simulink model "VBattery_harness"  (Simulink 7.7)
settings: Solver=FixedStepDiscrete  StartTime=0.0  StopTime=100.0  FixedStep=.1  RelTol=1e-3
PostLoadFcn:
  | load Vbattery.mat
InitFcn:
  | if signalbuilder('VBattery_harness/Signal_Builder','activegroup') == 1
  |   CD_VBATTERY_FUNCTION.DataType = 'uint8';
  |   CD_VBATTERY_FUNCTION.Value = 255;
  |   CD_ALTERNATOR_FUNCTION.DataType = 'uint8';
  |   CD_ALTERNATOR_FUNCTION.Value = 255;
  | elseif signalbuilder('VBattery_harness/Signal_Builder','activegroup') == 2
  |   CD_ALTERNATOR_FUNCTION.DataType = 'uint8';
  |   CD_ALTERNATOR_FUNCTION.Value = 255;
  |   CD_VBATTERY_FUNCTION.DataType = 'uint8';
  |   CD_VBATTERY_FUNCTION.Value = 0;
  | else
  |   CD_VBATTERY_FUNCTION.DataType = 'uint8';
  |   CD_VBATTERY_FUNCTION.Value = 0;
  |   CD_ALTERNATOR_FUNCTION.DataType = 'uint8';
  |   CD_ALTERNATOR_FUNCTION.Value = 0;
  | end
undefined symbols (not defined in the file): CD_PRECISION_REF_NOMINAL_VALUE, CD_VBATTERY_FILTER_DISPLAY_GAIN, CD_VBATTERY_FILTER_GAIN, CD_VBATTERY_GAIN, sigbuilder_block, srate100
settings Model: Creator=smindema  LastModifiedBy=aliebel  RecordCoverage=on  CovMetricSettings=dcw  CovCumulativeReport=on
settings DataIOCC: SaveFormat=Structure
settings OptimizationCC: InlineParams=on  InitFltsAndDblsToZero=on  EfficientFloat2IntCast=on  OptimizeModelRefInitCode=on
settings DebuggingCC: SaveWithParameterizedLinksMsg=none  SignalResolutionControl=TryResolveAllWithWarning  MultiTaskDSMMsg=warning  MultiTaskCondExecSysMsg=none  StrictBusMsg=Warning
settings HardwareCC: ProdBitPerInt=16  ProdBitPerPointer=16  ProdIntDivRoundTo=Floor  ProdEndianess=BigEndian  ProdWordSize=16  ProdHWDeviceType=Motorola HC12  TargetHWDeviceType=32-bit Generic  ProdEqTarget=off
settings RTWCC: SystemTargetFile=ert.tlc  GenCodeOnly=on  TemplateMakefile=ert_default_tmf  Description=Real-Time Workshop Embedded Coder (no auto configuration)  ProcessScript=ert_make_rtw_hook  IncludeERTFirstTime=on
settings CodeAppCC: IgnoreCustomStorageClasses=off
settings ERTTargetCC: TargetFcnLib=ansi_tfl_tmw.mat  FunctionExecutionProfile=off  MultiwordLength=2048  GenerateSampleERTMain=on  IncludeMdlTerminateFcn=off  SupportNonFinite=off  SupportComplex=off  PurelyIntegerCode=on  InlinedParameterPlacement=NonHierarchical  ERTCustomFileTemplate=example_file_process.tlc  ConvertIfToSwitch=off

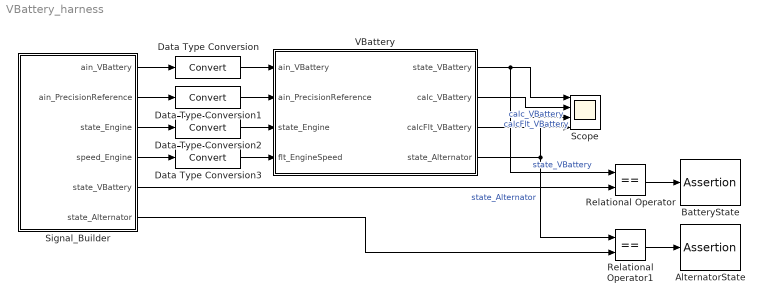
== system VBattery_harness ==
  AlternatorState : Assertion  Enabled=off
  BatteryState : Assertion  Enabled=off
  Data Type Conversion{,1..3} (4 alike) : DataTypeConversion
  Relational Operator : RelationalOperator  Operator===  OutDataTypeStr=boolean
  Relational Operator1 : RelationalOperator  Operator===  OutDataTypeStr=boolean
  Scope : Scope  NumInputPorts=4
      settings: TimeRange=100  YMin=8~14.5~14.5~8  YMax=11~21~21~10  MaxDataPoints=100000
  Signal_Builder : Subsystem  Tag=STV Subsys  LoadFcn=sigbuilder_block('load');  StartFcn=sigbuilder_block('start');  StopFcn=sigbuilder_block('stop');  ClipboardFcn=sigbuilder_block('clipboard');  mask(Sigbuilder block){}
      mask help: Sigbuilder GUI
      mask init:
      | if ~strcmp(get_param(bdroot(gcbh),'SimulationStatus'),'stopped') tuvar = sigbuilder_block('maskInit'); end
      settings: CopyFcn=sigbuilder_block('copy');  DeleteFcn=sigbuilder_block('delete');  ModelCloseFcn=sigbuilder_block('modelClose');  PreSaveFcn=sigbuilder_block('preSave');  NameChangeFcn=sigbuilder_block('namechange');  OpenFcn=sigbuilder_block('open',[50.25 223.5 1137 507 ]);  CloseFcn=sigbuilder_block('close');
      mask Display: plot(0,0,100,100,[10,10,40,40,10],[80,20,20,80,80],[40,10],[50,50], [40,27,10],[65,72,56],[40,25,25,10],[28,28,43,43]);
  VBattery : Subsystem  TreatAsAtomicUnit=on  SystemSampleTime=srate100  RTWFileName=mod_Inputs
      settings: RTWSystemCode=Function  RTWFcnNameOpts=Use subsystem name  RTWFileNameOpts=User specified
  wires:
  Signal_Builder/1(ain_VBattery) -> Data Type Conversion/1
  Data Type Conversion/1 -> VBattery/1(ain_VBattery)
  Data Type Conversion1/1 -> VBattery/2(ain_PrecisionReference)
  VBattery/1(state_VBattery) -> Scope/1, Relational Operator/1  "state_VBattery"
  VBattery/2(calc_VBattery) -> Scope/2  "calc_VBattery"
  VBattery/3(calcFlt_VBattery) -> Scope/3  "calcFlt_VBattery"
  Data Type Conversion2/1 -> VBattery/3(state_Engine)
  Signal_Builder/5(state_VBattery) -> Relational Operator/2
  Relational Operator/1 -> BatteryState/1
  Signal_Builder/4(speed_Engine) -> Data Type Conversion3/1
  Data Type Conversion3/1 -> VBattery/4(flt_EngineSpeed)
  Relational Operator1/1 -> AlternatorState/1
  VBattery/4(state_Alternator) -> Relational Operator1/1, Scope/4  "state_Alternator"
  Signal_Builder/6(state_Alternator) -> Relational Operator1/2
  Signal_Builder/2(ain_PrecisionReference) -> Data Type Conversion1/1
  Signal_Builder/3(state_Engine) -> Data Type Conversion2/1

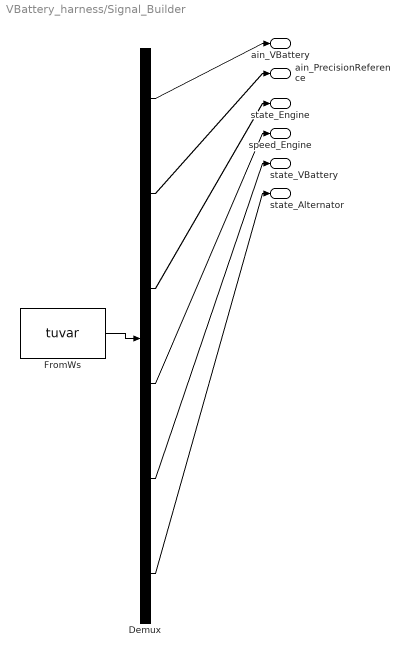
== system VBattery_harness/Signal_Builder ==
  Demux : Demux  Tag=STV Demux  Outputs=6
  FromWs : FromWorkspace  Tag=STV FromWs  VariableName=tuvar  SampleTime=0  SigBuilderData=DataTag0  VnvData=DataTag1
      SigBuilderData=|
      | common.afterFinalStr = 'Extrapolate'
      | common.sampleTime = 0
      | dataSet(1).timeRange = [0 100]
      | dataSet(1).name = 'T1-NONFUNC'
      | dataSet(2).timeRange = [0 100]
      | dataSet(2).name = 'T2-ALT NONFUNC'
      | dataSet(3).timeRange = [0 100]
      | dataSet(3).name = 'ALT_LOW'
      | dataSet(4).timeRange = [0 100]
      | dataSet(4).name = 'OORL'
      | dataSet(5).timeRange = [0 100]
      | dataSet(5).name = 'LOW'
      | dataSet(6).timeRange = [0 100]
      | dataSet(6).name = 'HIGH'
      | dataSet(7).timeRange = [0 100]
      | dataSet(7).name = 'NORMAL'
      | dataSet(8).timeRange = [0 100]
      | dataSet(8).name = 'HIGH2'
      | dataSet(9).timeRange = [0 100]
      | dataSet(9).name = 'HIGH3'
      | dataSet(10).timeRange = [0 100]
      | dataSet(10).name = 'ALT_HIGH'
      | sbobj.Groups(1).Name = 'T1-NONFUNC'
      | sbobj.Groups(1).Signals(1).Name = 'ain_VBattery'
      | sbobj.Groups(1).Signals(1).XData = [0 10 10 10.3 10.3 10.9 10.9 21.9 21.9 22.2 22.2 29.9 29.9 30.2 30.2 30.5 30.5 31.1 31.1 31.5 31.5 38.2 38.2 38.5 38.5 44 44 45.6 45.6 45.7 45.7 48 48 48.3 48.3 53.5 53.5 53.7 53.7 60 60 66.4 66.4 69.9 69.9 79.8 79.8 89.9 89.9 100]
      | sbobj.Groups(1).Signals(1).YData = [500 500 298 298 500 500 298 298 500 500 298 298 226 226 500 500 226 226 300 300 226 226 390 332 226 226 500 500 226 226 500 500 300 300 500 500 300 300 500 500 296 296 502 502 224 224 298 298 500 500]
      | sbobj.Groups(1).Signals(2).Name = 'ain_PrecisionReference'
      | sbobj.Groups(1).Signals(2).XData = [0 100]
      | sbobj.Groups(1).Signals(2).YData = [509 509]
      | sbobj.Groups(1).Signals(3).Name = 'state_Engine'
      | sbobj.Groups(1).Signals(3).XData = [0 50 50 100]
      | sbobj.Groups(1).Signals(3).YData = [1 1 2 2]
      | sbobj.Groups(1).Signals(4).Name = 'speed_Engine'
      | sbobj.Groups(1).Signals(4).XData = [0 8.6 8.6 53.2 53.2 65.2 65.2 100]
      | sbobj.Groups(1).Signals(4).YData = [0 0 1500 1500 0 0 1500 1500]
      | sbobj.Groups(1).Signals(5).Name = 'state_VBattery'
      | sbobj.Groups(1).Signals(5).XData = [0 100]
      | sbobj.Groups(1).Signals(5).YData = [8 8]
      | sbobj.Groups(1).Signals(6).Name = 'state_Alternator'
      | sbobj.Groups(1).Signals(6).XData = [0 100]
      | sbobj.Groups(1).Signals(6).YData = [8 8]
      | sbobj.Groups(2).Name = 'T2-ALT NONFUNC'
      | sbobj.Groups(2).Signals(1).Name = 'ain_VBattery'
      | sbobj.Groups(2).Signals(1).XData = [0 10 10 10.3 10.3 10.9 10.9 21.9 21.9 22.2 22.2 29.9 29.9 30.2 30.2 30.5 30.5 31.1 31.1 31.5 31.5 38.2 38.2 38.5 38.5 45.9 47.4 47.4 53.5 53.5 53.7 53.7 60 60 66.4 66.4 69.9 69.9 79.8 79.8 89.9 89.9 100]
      | sbobj.Groups(2).Signals(1).YData = [500 500 298 298 500 500 298 298 500 500 298 298 226 226 500 500 226 226 300 300 226 226 390 332 300 300 300 630 630 300 300 595 595 296 296 502 502 224 224 298 298 500 500]
      | sbobj.Groups(2).Signals(2).Name = 'ain_PrecisionReference'
      | sbobj.Groups(2).Signals(2).XData = [0 100]
      | sbobj.Groups(2).Signals(2).YData = [509 509]
      | sbobj.Groups(2).Signals(3).Name = 'state_Engine'
      | sbobj.Groups(2).Signals(3).XData = [0 50 50 100]
      | sbobj.Groups(2).Signals(3).YData = [1 1 2 2]
      | sbobj.Groups(2).Signals(4).Name = 'speed_Engine'
      | sbobj.Groups(2).Signals(4).XData = [0 8.6 8.6 34.8 35.2 53.2 53.2 65.2 65.2 100]
      | sbobj.Groups(2).Signals(4).YData = [0 0 1500 1500 1500 1500 0 0 1500 1500]
      | sbobj.Groups(2).Signals(5).Name = 'state_VBattery'
      | sbobj.Groups(2).Signals(5).XData = [0 12.4 12.4 32.2 32.2 38.9 38.9 48 48 48.9 48.9 55.6 60.6 60.6 61.9 61.9 71.7 71.7 100]
      | sbobj.Groups(2).Signals(5).YData = [8 8 9 9 14 14 9 9 8 8 10 10 10 8 8 9 9 14 14]
      | sbobj.Groups(2).Signals(6).Name = 'state_Alternator'
      | sbobj.Groups(2).Signals(6).XData = [0 100]
      | sbobj.Groups(2).Signals(6).YData = [8 8]
      | sbobj.Groups(3).Name = 'ALT_LOW'
      | sbobj.Groups(3).Signals(1).Name = 'ain_VBattery'
      | sbobj.Groups(3).Signals(1).XData = [0 10 10 10.3 10.3 10.9 10.9 21.9 21.9 22.2 22.2 29.9 29.9 30.2 30.2 30.5 30.5 31.1 31.1 31.5 31.5 38.2 38.2 38.5 38.5 42.4 42.4 53.1 53.1 53.5 53.5 53.7 53.7 60 60 66.4 66.4 69.9 69.9 79.8 79.8 89.9 89.9 100]
      | sbobj.Groups(3).Signals(1).YData = [500 500 298 298 500 500 298 298 500 500 298 298 226 226 500 500 226 226 300 300 226 226 390 332 226 226 360 360 500 500 300 300 500 500 296 296 502 502 224 224 298 298 500 500]
      | sbobj.Groups(3).Signals(2).Name = 'ain_PrecisionReference'
      | sbobj.Groups(3).Signals(2).XData = [0 100]
      | sbobj.Groups(3).Signals(2).YData = [509 509]
      | sbobj.Groups(3).Signals(3).Name = 'state_Engine'
      | sbobj.Groups(3).Signals(3).XData = [0 50 50 70 70 100]
      | sbobj.Groups(3).Signals(3).YData = [1 1 2 2 3 3]
      | sbobj.Groups(3).Signals(4).Name = 'speed_Engine'
      | sbobj.Groups(3).Signals(4).XData = [0 8.6 8.6 22.7 22.7 26.6 26.6 42 42 47.3 47.3 53.2 53.2 69 69 100]
      | sbobj.Groups(3).Signals(4).YData = [0 0 1500 1500 20 20 1500 1500 0 0 1500 1500 0 0 1500 1500]
      | sbobj.Groups(3).Signals(5).Name = 'state_VBattery'
      | sbobj.Groups(3).Signals(5).XData = [0 12.4 23.3 23.3 32.2 32.2 43.2 43.2 45.7 45.7 61.6 61.6 70.7 70.7 71.7 71.7 81 81 100]
      | sbobj.Groups(3).Signals(5).YData = [8 8 8 9 9 14 14 9 9 8 8 9 9 8 8 14 14 8 8]
      | sbobj.Groups(3).Signals(6).Name = 'state_Alternator'
      | sbobj.Groups(3).Signals(6).XData = [0 11.7 11.7 23.3 23.3 47.8 47.8 53.7 53.7 70.7 70.7 71.7 71.7 81 81 91.1 91.1 100]
      | sbobj.Groups(3).Signals(6).YData = [8 8 9 9 8 8 9 9 8 8 9 9 8 8 9 9 8 8]
      | sbobj.Groups(4).Name = 'OORL'
      | sbobj.Groups(4).Signals(1).Name = 'ain_VBattery'
      | sbobj.Groups(4).Signals(1).XData = [0 29.9 29.9 30.6 30.6 40 40 48.3 48.3 52.2 52.2 78 78 87 87 94 94 94.7 94.7 100]
      | sbobj.Groups(4).Signals(1).YData = [500 500 0 0 500 500 4 4 495 495 34 34 500 500 38 38 500 500 38 38]
      | sbobj.Groups(4).Signals(2).Name = 'ain_PrecisionReference'
      | sbobj.Groups(4).Signals(2).XData = [0 100]
      | sbobj.Groups(4).Signals(2).YData = [509 509]
      | sbobj.Groups(4).Signals(3).Name = 'state_Engine'
      | sbobj.Groups(4).Signals(3).XData = [0 37.6 37.6 67.6 67.6 100]
      | sbobj.Groups(4).Signals(3).YData = [1 1 2 2 1 1]
      | sbobj.Groups(4).Signals(4).Name = 'speed_Engine'
      | sbobj.Groups(4).Signals(4).XData = [0 100]
      | sbobj.Groups(4).Signals(4).YData = [0 0]
      | sbobj.Groups(4).Signals(5).Name = 'state_VBattery'
      | sbobj.Groups(4).Signals(5).XData = [0 41.1 41.1 79.3 79.3 88.2 88.2 100]
      | sbobj.Groups(4).Signals(5).YData = [8 8 22 22 8 8 22 22]
      | sbobj.Groups(4).Signals(6).Name = 'state_Alternator'
      | sbobj.Groups(4).Signals(6).XData = [0 100]
      | sbobj.Groups(4).Signals(6).YData = [8 8]
      | sbobj.Groups(5).Name = 'LOW'
      | sbobj.Groups(5).Signals(1).Name = 'ain_VBattery'
      | sbobj.Groups(5).Signals(1).XData = [0 10 10 10.3 10.3 10.9 10.9 21.9 21.9 22.2 22.2 29.9 29.9 30.2 30.2 30.5 30.5 31.1 31.1 31.5 31.5 38.2 38.2 38.5 38.5 44 44 45.6 45.6 45.7 45.7 48 48 48.3 48.3 53.5 53.5 53.7 53.7 60 60 66.4 66.4 69.9 69.9 79.8 79.8 89.9 89.9 100]
      | sbobj.Groups(5).Signals(1).YData = [500 500 298 298 500 500 298 298 500 500 298 298 226 226 500 500 226 226 300 300 226 226 390 332 226 226 500 500 226 226 500 500 300 300 500 500 300 300 500 500 296 296 502 502 224 224 298 298 500 500]
      | sbobj.Groups(5).Signals(2).Name = 'ain_PrecisionReference'
      | sbobj.Groups(5).Signals(2).XData = [0 100]
      | sbobj.Groups(5).Signals(2).YData = [509 509]
      | sbobj.Groups(5).Signals(3).Name = 'state_Engine'
      | sbobj.Groups(5).Signals(3).XData = [0 50 50 100]
      | sbobj.Groups(5).Signals(3).YData = [1 1 2 2]
      | sbobj.Groups(5).Signals(4).Name = 'speed_Engine'
      | sbobj.Groups(5).Signals(4).XData = [0 91.7 91.7 92 92 100]
      | sbobj.Groups(5).Signals(4).YData = [0 0 1600 1600 0 0]
      | sbobj.Groups(5).Signals(5).Name = 'state_VBattery'
      | sbobj.Groups(5).Signals(5).XData = [0 12.4 12.4 32.2 32.2 44.9 44.9 61.6 61.6 71.7 71.7 83.4 86.3 92.3 92.3 100]
      | sbobj.Groups(5).Signals(5).YData = [8 8 9 9 14 14 8 8 9 9 14 14 14 14 8 8]
      | sbobj.Groups(5).Signals(6).Name = 'state_Alternator'
      | sbobj.Groups(5).Signals(6).XData = [0 100]
      | sbobj.Groups(5).Signals(6).YData = [8 8]
      | sbobj.Groups(6).Name = 'HIGH'
      | sbobj.Groups(6).Signals(1).Name = 'ain_VBattery'
      | sbobj.Groups(6).Signals(1).XData = [0 10 10 10.3 10.3 10.9 10.9 16 16 16.5 16.5 21.9 21.9 22.2 22.2 29.9 29.9 30.2 30.2 30.4 30.4 30.7 30.7 30.9 30.9 38 38 38.1 38.1 44 44 45.6 45.6 45.7 45.7 48 48 48.3 48.3 53.5 53.5 53.7 53.7 60 60 69.9 69.9 79.8 79.8 89.9 89.9 100]
      | sbobj.Groups(6).Signals(1).YData = [500 500 630 630 500 500 570 570 738 738 570 570 500 500 572 572 700 700 500 500 700 700 625 625 700 700 500 500 700 700 500 500 700 700 500 500 620 625 500 500 630 630 500 500 562 562 700 700 556 556 500 500]
      | sbobj.Groups(6).Signals(2).Name = 'ain_PrecisionReference'
      | sbobj.Groups(6).Signals(2).XData = [0 100]
      | sbobj.Groups(6).Signals(2).YData = [509 509]
      | sbobj.Groups(6).Signals(3).Name = 'state_Engine'
      | sbobj.Groups(6).Signals(3).XData = [0 50 50 100]
      | sbobj.Groups(6).Signals(3).YData = [1 1 2 2]
      | sbobj.Groups(6).Signals(4).Name = 'speed_Engine'
      | sbobj.Groups(6).Signals(4).XData = [0 100]
      | sbobj.Groups(6).Signals(4).YData = [0 0]
      | sbobj.Groups(6).Signals(5).Name = 'state_VBattery'
      | sbobj.Groups(6).Signals(5).XData = [0 11.8 11.8 32.3 32.3 44.6 44.6 46.5 46.5 61.4 61.4 71.8 71.8 80.5 80.5 90.9 90.9 100]
      | sbobj.Groups(6).Signals(5).YData = [8 8 10 10 11 11 10 10 8 8 10 10 11 11 10 10 8 8]
      | sbobj.Groups(6).Signals(6).Name = 'state_Alternator'
      | sbobj.Groups(6).Signals(6).XData = [0 100]
      | sbobj.Groups(6).Signals(6).YData = [8 8]
      | sbobj.Groups(7).Name = 'NORMAL'
      | sbobj.Groups(7).Signals(1).Name = 'ain_VBattery'
      | sbobj.Groups(7).Signals(1).XData = [0 100]
      | sbobj.Groups(7).Signals(1).YData = [498 498]
      | sbobj.Groups(7).Signals(2).Name = 'ain_PrecisionReference'
      | sbobj.Groups(7).Signals(2).XData = [0 100]
      | sbobj.Groups(7).Signals(2).YData = [509 509]
      | sbobj.Groups(7).Signals(3).Name = 'state_Engine'
      | sbobj.Groups(7).Signals(3).XData = [0 50 50 100]
      | sbobj.Groups(7).Signals(3).YData = [1 1 2 2]
      | sbobj.Groups(7).Signals(4).Name = 'speed_Engine'
      | sbobj.Groups(7).Signals(4).XData = [0 100]
      | sbobj.Groups(7).Signals(4).YData = [0 0]
      | sbobj.Groups(7).Signals(5).Name = 'state_VBattery'
      | sbobj.Groups(7).Signals(5).XData = [0 100]
      | sbobj.Groups(7).Signals(5).YData = [8 8]
      | sbobj.Groups(7).Signals(6).Name = 'state_Alternator'
      | sbobj.Groups(7).Signals(6).XData = [0 100]
      | sbobj.Groups(7).Signals(6).YData = [8 8]
      | sbobj.Groups(8).Name = 'HIGH2'
      | sbobj.Groups(8).Signals(1).Name = 'ain_VBattery'
      | sbobj.Groups(8).Signals(1).XData = [0 20 20 60 60 100]
      | sbobj.Groups(8).Signals(1).YData = [498 498 610 610 0 0]
      | sbobj.Groups(8).Signals(2).Name = 'ain_PrecisionReference'
      | sbobj.Groups(8).Signals(2).XData = [0 100]
      | sbobj.Groups(8).Signals(2).YData = [509 509]
      | sbobj.Groups(8).Signals(3).Name = 'state_Engine'
      | sbobj.Groups(8).Signals(3).XData = [0 50 50 100]
      | sbobj.Groups(8).Signals(3).YData = [1 1 2 2]
      | sbobj.Groups(8).Signals(4).Name = 'speed_Engine'
      | sbobj.Groups(8).Signals(4).XData = [0 100]
      | sbobj.Groups(8).Signals(4).YData = [0 0]
      | sbobj.Groups(8).Signals(5).Name = 'state_VBattery'
      | sbobj.Groups(8).Signals(5).XData = [0 20.8 20.8 61.3 61.3 100]
      | sbobj.Groups(8).Signals(5).YData = [8 8 10 10 22 22]
      | sbobj.Groups(8).Signals(6).Name = 'state_Alternator'
      | sbobj.Groups(8).Signals(6).XData = [0 100]
      | sbobj.Groups(8).Signals(6).YData = [8 8]
      | sbobj.Groups(9).Name = 'HIGH3'
      | sbobj.Groups(9).Signals(1).Name = 'ain_VBattery'
      | sbobj.Groups(9).Signals(1).XData = [0 10 10 10.3 10.3 10.9 10.9 16 16 16.5 16.5 21.9 21.9 22.2 22.2 29.9 29.9 30.2 30.2 30.4 30.4 30.7 30.7 30.9 30.9 38 38 38.8 38.8 44 44 45.6 45.6 45.7 45.7 48 48 48.3 48.3 53.5 53.5 53.7 53.7 60 60 69.9 69.9 79.8 79.8 83 83 100]
      | sbobj.Groups(9).Signals(1).YData = [500 500 630 630 500 500 580 580 738 738 580 580 500 500 580 580 700 700 500 500 700 700 625 625 700 700 640 645 700 700 500 500 700 700 500 500 620 625 500 500 630 630 500 500 575 575 700 700 575 575 500 500]
      | sbobj.Groups(9).Signals(2).Name = 'ain_PrecisionReference'
      | sbobj.Groups(9).Signals(2).XData = [0 100]
      | sbobj.Groups(9).Signals(2).YData = [509 509]
      | sbobj.Groups(9).Signals(3).Name = 'state_Engine'
      | sbobj.Groups(9).Signals(3).XData = [0 50 50 100]
      | sbobj.Groups(9).Signals(3).YData = [1 1 2 2]
      | sbobj.Groups(9).Signals(4).Name = 'speed_Engine'
      | sbobj.Groups(9).Signals(4).XData = [0 100]
      | sbobj.Groups(9).Signals(4).YData = [0 0]
      | sbobj.Groups(9).Signals(5).Name = 'state_VBattery'
      | sbobj.Groups(9).Signals(5).XData = [0 11.7 11.7 32.3 32.3 44.6 44.6 46.5 46.5 61.1 61.1 71.7 71.7 80.5 80.5 84.2 84.2 100]
      | sbobj.Groups(9).Signals(5).YData = [8 8 10 10 11 11 10 10 8 8 10 10 11 11 10 10 8 8]
      | sbobj.Groups(9).Signals(6).Name = 'state_Alternator'
      | sbobj.Groups(9).Signals(6).XData = [0 100]
      | sbobj.Groups(9).Signals(6).YData = [8 8]
      | sbobj.Groups(10).Name = 'ALT_HIGH'
      | sbobj.Groups(10).Signals(1).Name = 'ain_VBattery'
      | sbobj.Groups(10).Signals(1).XData = [0 10 10 10.3 10.3 10.9 10.9 16 16 16.3 16.3 21.9 21.9 22.2 22.2 29.9 29.9 30.2 30.2 30.4 30.4 30.7 30.7 30.9 30.9 38 38 39 39 44 44 45.6 45.6 45.7 45.7 48 48 48.3 48.3 53.5 53.5 53.7 53.7 60 60 69.9 69.9 79.8 79.8 89.9 89.9 100]
      | sbobj.Groups(10).Signals(1).YData = [500 500 630 630 500 500 585 585 738 738 585 585 500 500 585 585 700 700 500 500 700 700 625 625 700 700 500 500 700 700 500 500 700 700 500 500 620 625 500 500 630 630 500 500 580 580 700 700 580 580 500 500]
      | sbobj.Groups(10).Signals(2).Name = 'ain_PrecisionReference'
      | sbobj.Groups(10).Signals(2).XData = [0 100]
      | sbobj.Groups(10).Signals(2).YData = [509 509]
      | sbobj.Groups(10).Signals(3).Name = 'state_Engine'
      | sbobj.Groups(10).Signals(3).XData = [0 50 50 100]
      | sbobj.Groups(10).Signals(3).YData = [1 1 2 2]
      | sbobj.Groups(10).Signals(4).Name = 'speed_Engine'
      | sbobj.Groups(10).Signals(4).XData = [0 15 15 25 25 33.2 33.2 100]
      | sbobj.Groups(10).Signals(4).YData = [0 0 1500 1500 540 540 1500 1500]
      | sbobj.Groups(10).Signals(5).Name = 'state_VBattery'
      | sbobj.Groups(10).Signals(5).XData = [0 11.7 11.7 32.3 32.3 38.5 38.5 40.9 40.9 44.5 44.5 71.7 71.7 80.4 80.4 91.2 100]
      | sbobj.Groups(10).Signals(5).YData = [8 8 10 10 11 11 8 8 11 11 8 8 11 11 8 8 8]
      | sbobj.Groups(10).Signals(6).Name = 'state_Alternator'
      | sbobj.Groups(10).Signals(6).XData = [0 38.5 38.5 40.9 40.9 44.5 44.5 46.5 46.5 60.9 60.9 71.7 71.7 80.4 80.4 91.2 91.2 100]
      | sbobj.Groups(10).Signals(6).YData = [8 8 10 10 8 8 10 10 8 8 10 10 8 8 10 10 8 8]
  ain_VBattery : Outport  Tag=STV Outport
  ain_PrecisionReference : Outport  Tag=STV Outport  Port=2
  state_Engine : Outport  Tag=STV Outport  Port=3
  speed_Engine : Outport  Tag=STV Outport  Port=4
  state_VBattery : Outport  Tag=STV Outport  Port=5
  state_Alternator : Outport  Tag=STV Outport  Port=6
  wires:
  FromWs/1 -> Demux/1
  Demux/1 -> ain_VBattery/1
  Demux/2 -> ain_PrecisionReference/1
  Demux/3 -> state_Engine/1
  Demux/4 -> speed_Engine/1
  Demux/5 -> state_VBattery/1
  Demux/6 -> state_Alternator/1

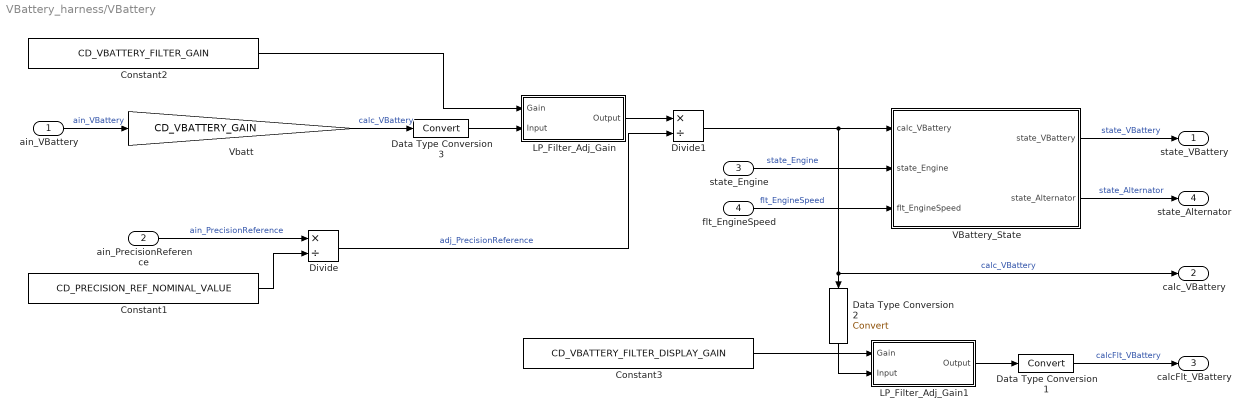
== system VBattery_harness/VBattery ==
  ain_VBattery : Inport  OutDataTypeStr=uint16
  ain_PrecisionReference : Inport  Port=2  OutDataTypeStr=uint16
  state_Engine : Inport  Port=3
  flt_EngineSpeed : Inport  Port=4  OutDataTypeStr=uint16
  Constant1 : Constant  Value=CD_PRECISION_REF_NOMINAL_VALUE  OutDataTypeStr=uint16  SampleTime=srate100
  Constant2 : Constant  Value=CD_VBATTERY_FILTER_GAIN  OutDataTypeStr=uint8  SampleTime=srate100
  Constant3 : Constant  Value=CD_VBATTERY_FILTER_DISPLAY_GAIN  OutDataTypeStr=uint8  SampleTime=srate100
  Data Type Conversion1 : DataTypeConversion
  Data Type Conversion2 : DataTypeConversion
  Data Type Conversion3 : DataTypeConversion
  Divide : Product  Inputs=*/  OutDataTypeStr=fixdt(0,16,10)  RndMeth=Nearest
  Divide1 : Product  Inputs=*/  OutDataTypeStr=fixdt(0,16,8)  RndMeth=Nearest
  LP_Filter_Adj_Gain : Subsystem
  LP_Filter_Adj_Gain1 : Subsystem
  VBattery_State : Stateflow chart  TreatAsAtomicUnit=on
  Vbatt : Gain  Gain=CD_VBATTERY_GAIN  ParamDataTypeStr=fixdt(0,16,12)  OutDataTypeStr=fixdt(0,16,8)  RndMeth=Nearest  SampleTime=srate100  SaturateOnIntegerOverflow=on
  state_VBattery : Outport  OutDataTypeStr=uint8
  calc_VBattery : Outport  Port=2
  calcFlt_VBattery : Outport  Port=3  OutDataTypeStr=fixdt(0,16,8)
  state_Alternator : Outport  Port=4  OutDataTypeStr=uint8
  wires:
  ain_VBattery/1 -> Vbatt/1  "ain_VBattery"
  state_Engine/1 -> VBattery_State/2(state_Engine)  "state_Engine"
  Data Type Conversion1/1 -> calcFlt_VBattery/1  "calcFlt_VBattery"
  LP_Filter_Adj_Gain1/1(Output) -> Data Type Conversion1/1
  ain_PrecisionReference/1 -> Divide/1  "ain_PrecisionReference"
  Constant1/1 -> Divide/2
  Divide/1 -> Divide1/2  "adj_PrecisionReference"
  Vbatt/1 -> Data Type Conversion3/1  "calc_VBattery"
  Divide1/1 -> VBattery_State/1(calc_VBattery), calc_VBattery/1, Data Type Conversion2/1  "calc_VBattery"
  LP_Filter_Adj_Gain/1(Output) -> Divide1/1
  flt_EngineSpeed/1 -> VBattery_State/3(flt_EngineSpeed)  "flt_EngineSpeed"
  VBattery_State/1(state_VBattery) -> state_VBattery/1  "state_VBattery"
  VBattery_State/2(state_Alternator) -> state_Alternator/1  "state_Alternator"
  Constant2/1 -> LP_Filter_Adj_Gain/1(Gain)
  Constant3/1 -> LP_Filter_Adj_Gain1/1(Gain)
  Data Type Conversion2/1 -> LP_Filter_Adj_Gain1/2(Input)
  Data Type Conversion3/1 -> LP_Filter_Adj_Gain/2(Input)

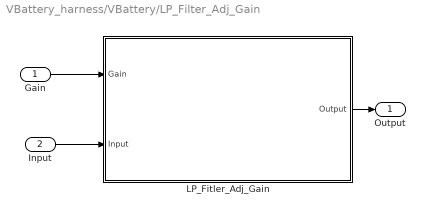
== system VBattery_harness/VBattery/LP_Filter_Adj_Gain ==
  Gain : Inport
  Input : Inport  Port=2
  LP_Fitler_Adj_Gain : Stateflow chart  TreatAsAtomicUnit=on
  Output : Outport
  wires:
  LP_Fitler_Adj_Gain/1(Output) -> Output/1
  Input/1 -> LP_Fitler_Adj_Gain/2(Input)
  Gain/1 -> LP_Fitler_Adj_Gain/1(Gain)

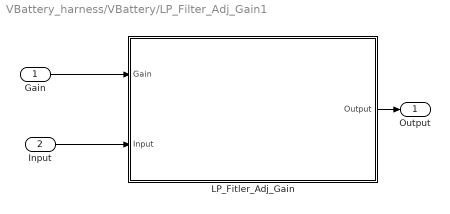
== system VBattery_harness/VBattery/LP_Filter_Adj_Gain1 ==
  Gain : Inport
  Input : Inport  Port=2
  LP_Fitler_Adj_Gain : Stateflow chart  TreatAsAtomicUnit=on
  Output : Outport
  wires:
  LP_Fitler_Adj_Gain/1(Output) -> Output/1
  Input/1 -> LP_Fitler_Adj_Gain/2(Input)
  Gain/1 -> LP_Fitler_Adj_Gain/1(Gain)

== stateflow chart VBattery/LP_Filter_Adj_Gain/LP_Fitler_Adj_Gain ==
  state INITIAL
    en:Output = Input;
  state LP_FILTER
    du:Output = Output + ((Input - Output)/(1 << Gain));
  (default) -> INITIAL
  INITIAL -> LP_FILTER
  data: Gain input uint8; Input input fixdt(1,16,8); Output output fixdt(1,32,16)

== stateflow chart VBattery/VBattery_State ==
  state NON_FUNCTIONAL
    en:state_VBattery = NORMAL;
    en:state_Alternator = NORMAL;
  state NORMAL
    state NORMAL
      state NORMAL
        en:state_VBattery = NORMAL;
        en:state_Alternator = NORMAL;
      state DEBOUNCE
        en:debounceCount = 0;
        du:debounceCount++;
      (default) -> NORMAL.NORMAL.DEBOUNCE
      NORMAL.NORMAL.DEBOUNCE -> NORMAL.NORMAL.NORMAL : [(debounceCount >= CD_VBATTERY_DEBOUNCE_NORMAL)...
          | || ((state_VBattery == NORMAL) && (state_Alternator == NORMAL))]
    state HIGH
      state HIGH
        en:state_VBattery = HIGH;
        en:state_Alternator = NORMAL;
      state DEBOUNCE
        en:debounceCount = 0;
        du:debounceCount++;
      NORMAL.HIGH.DEBOUNCE -> NORMAL.HIGH.HIGH : [(debounceCount >= CD_VBATTERY_DEBOUNCE_HIGH)...
          | || (state_VBattery == HIGH)]
      (default) -> NORMAL.HIGH.DEBOUNCE
    state EXTREMELY_LOW
      state DEBOUNCE
        en:debounceCount = 0;
        du:debounceCount++;
      state EXTREMELY_LOW
        en:state_VBattery = EXTREMELY_LOW;
        en:state_Alternator = NORMAL;
      NORMAL.EXTREMELY_LOW.DEBOUNCE -> NORMAL.EXTREMELY_LOW.EXTREMELY_LOW : [(debounceCount >= CD_VBATTERY_DEBOUNCE_EXTREMELY_LOW)...
          | || (state_VBattery == EXTREMELY_LOW)]
      (default) -> NORMAL.EXTREMELY_LOW.DEBOUNCE
    state LOW
      state LOW
        en:state_VBattery = LOW;
        en:state_Alternator = NORMAL;
      state DEBOUNCE
        en:debounceCount = 0;
        du:debounceCount++;
      NORMAL.LOW.DEBOUNCE -> NORMAL.LOW.LOW : [(debounceCount >= CD_VBATTERY_DEBOUNCE_LOW)...
          | || (state_VBattery == LOW)]
      (default) -> NORMAL.LOW.DEBOUNCE
    state EXTREMELY_HIGH
      state DEBOUNCE
        en:debounceCount = 0;
        du:debounceCount++;
      state EXTREMELY_HIGH
        en:state_VBattery = EXTREMELY_HIGH;
        en:state_Alternator = NORMAL;
      NORMAL.EXTREMELY_HIGH.DEBOUNCE -> NORMAL.EXTREMELY_HIGH.EXTREMELY_HIGH : [(debounceCount >= CD_VBATTERY_DEBOUNCE_EXTREMELY_HIGH)...
          | || (state_VBattery == EXTREMELY_HIGH)]
      (default) -> NORMAL.EXTREMELY_HIGH.DEBOUNCE
    state ALTERNATOR_LOW
      state DEBOUNCE
        en:debounceCount = 0;
        du:debounceCount++;
      state LOW
        en:state_Alternator = LOW;
        en:state_VBattery = NORMAL;
      (default) -> NORMAL.ALTERNATOR_LOW.DEBOUNCE
      NORMAL.ALTERNATOR_LOW.DEBOUNCE -> NORMAL.ALTERNATOR_LOW.LOW : [(debounceCount >= CD_ALTERNATOR_DEBOUNCE_LOW)]
    state ALTERNATOR_HIGH
      state DEBOUNCE
        en:debounceCount = 0;
        du:debounceCount++;
      state HIGH
        en:state_Alternator = HIGH;
        en:state_VBattery = NORMAL;
      (default) -> NORMAL.ALTERNATOR_HIGH.DEBOUNCE
      NORMAL.ALTERNATOR_HIGH.DEBOUNCE -> NORMAL.ALTERNATOR_HIGH.HIGH : [(debounceCount >= CD_ALTERNATOR_DEBOUNCE_HIGH)]
    NORMAL.EXTREMELY_HIGH -> NORMAL.HIGH [order 2] : [(calc_VBattery < (CD_VBATTERY_EXTREMELY_HIGH - CD_VOLTAGE_HYSTERESIS))...
        | && ((CD_ALTERNATOR_FUNCTION ==NON_FUNCTIONAL)...
        |   || (flt_EngineSpeed < CD_ALTERNATOR_ALARM_ENGINE_SPEED))]
    NORMAL.HIGH -> NORMAL.EXTREMELY_HIGH [order 1] : [(calc_VBattery >= CD_VBATTERY_EXTREMELY_HIGH)]
    (default) -> NORMAL.NORMAL
    NORMAL.HIGH -> NORMAL.NORMAL [order 2] : [(calc_VBattery < (CD_VBATTERY_HIGH - CD_VOLTAGE_HYSTERESIS))]
    NORMAL.NORMAL -> NORMAL.HIGH [order 3] : [(calc_VBattery >= CD_VBATTERY_HIGH)...
        | && ((CD_ALTERNATOR_FUNCTION ==NON_FUNCTIONAL)...
        |    ||  (flt_EngineSpeed < CD_ALTERNATOR_ALARM_ENGINE_SPEED))]
    NORMAL.NORMAL -> NORMAL.LOW [order 4] : [(calc_VBattery <= CD_VBATTERY_LOW)...
        | && ((CD_ALTERNATOR_FUNCTION == NON_FUNCTIONAL)...
        |   ||  (flt_EngineSpeed < CD_ALTERNATOR_ALARM_ENGINE_SPEED))]
    NORMAL.LOW -> NORMAL.NORMAL [order 1] : [(calc_VBattery > (CD_VBATTERY_LOW + CD_VOLTAGE_HYSTERESIS))...
        | && (state_Engine != ENGINE_CRANKING)]
    NORMAL.LOW -> NORMAL.EXTREMELY_LOW [order 2] : [(calc_VBattery <= CD_VBATTERY_EXTREMELY_LOW)]
    NORMAL.EXTREMELY_LOW -> NORMAL.LOW [order 2] : [(calc_VBattery > (CD_VBATTERY_EXTREMELY_LOW + CD_VOLTAGE_HYSTERESIS))...
        | && (state_Engine != ENGINE_CRANKING)...
        | && ((CD_ALTERNATOR_FUNCTION == NON_FUNCTIONAL)...
        |   ||  (flt_EngineSpeed < CD_ALTERNATOR_ALARM_ENGINE_SPEED))]
    NORMAL.NORMAL -> ALTERNATOR_LOW [order 1] : [(CD_ALTERNATOR_FUNCTION != NON_FUNCTIONAL)...
        | && (calc_VBattery <= CD_ALTERNATOR_LOW)...
        | && (flt_EngineSpeed >= CD_ALTERNATOR_ALARM_ENGINE_SPEED)]
    ALTERNATOR_LOW -> NORMAL.NORMAL [order 1] : [(calc_VBattery > (CD_ALTERNATOR_LOW + CD_VOLTAGE_HYSTERESIS))...
        | || (flt_EngineSpeed < CD_ALTERNATOR_ALARM_ENGINE_SPEED)]
    NORMAL.NORMAL -> ALTERNATOR_HIGH [order 2] : [(CD_ALTERNATOR_FUNCTION != NON_FUNCTIONAL)...
        | && (calc_VBattery >= CD_ALTERNATOR_HIGH)...
        | && (flt_EngineSpeed >= CD_ALTERNATOR_ALARM_ENGINE_SPEED)]
    ALTERNATOR_HIGH -> NORMAL.NORMAL [order 1] : [(calc_VBattery < (CD_ALTERNATOR_HIGH - CD_VOLTAGE_HYSTERESIS))...
        | || (flt_EngineSpeed < CD_ALTERNATOR_ALARM_ENGINE_SPEED)]
    NORMAL.EXTREMELY_LOW -> ALTERNATOR_LOW [order 1] : [(calc_VBattery > (CD_VBATTERY_EXTREMELY_LOW + CD_VOLTAGE_HYSTERESIS))...
        | && ((CD_ALTERNATOR_FUNCTION != NON_FUNCTIONAL) && (flt_EngineSpeed >= CD_ALTERNATOR_ALARM_ENGINE_SPEED))]
    ALTERNATOR_LOW -> NORMAL.EXTREMELY_LOW [order 2] : [(calc_VBattery <= CD_VBATTERY_EXTREMELY_LOW)]
    ALTERNATOR_HIGH -> NORMAL.EXTREMELY_HIGH [order 2] : [(calc_VBattery >= CD_VBATTERY_EXTREMELY_HIGH)]
    NORMAL.EXTREMELY_HIGH -> ALTERNATOR_HIGH [order 1] : [(calc_VBattery < (CD_VBATTERY_EXTREMELY_HIGH - CD_VOLTAGE_HYSTERESIS))...
        | && ((CD_ALTERNATOR_FUNCTION != NON_FUNCTIONAL) && (flt_EngineSpeed >= CD_ALTERNATOR_ALARM_ENGINE_SPEED))]
  state OORL
    state DEBOUNCE_OORL
      en:debounceCount = 0;
      du:debounceCount++;
    state OORL
      en:state_VBattery = OORL;
      en:state_Alternator = NORMAL;
    DEBOUNCE_OORL -> OORL.OORL : [(debounceCount >= CD_VBATTERY_DEBOUNCE_OORL)...
        | || (state_VBattery == OORL)]
    (default) -> DEBOUNCE_OORL
  (default) -> NON_FUNCTIONAL
  NORMAL -> OORL : [(calc_VBattery <= CD_VBATTERY_OORL)]
  OORL -> NORMAL : [(state_Engine != ENGINE_CRANKING)...
      | && (calc_VBattery > (CD_VBATTERY_OORL + CD_VOLTAGE_HYSTERESIS))]
  NON_FUNCTIONAL -> NORMAL : [(CD_VBATTERY_FUNCTION != NON_FUNCTIONAL)]
  data: state_VBattery output uint8; calc_VBattery input fixdt(0,16,8); debounceCount local uint16 =0; CD_VBATTERY_DEBOUNCE_EXTREMELY_LOW parameter uint16; CD_VBATTERY_DEBOUNCE_HIGH parameter uint16; CD_VBATTERY_DEBOUNCE_LOW parameter uint16; CD_VBATTERY_DEBOUNCE_NORMAL parameter uint16; CD_VBATTERY_DEBOUNCE_OORL parameter uint16; CD_VBATTERY_EXTREMELY_LOW parameter uint16; CD_VBATTERY_FUNCTION parameter uint8; CD_VBATTERY_HIGH parameter uint8; CD_VBATTERY_LOW parameter uint8; CD_VBATTERY_OORL parameter uint8; state_Engine input uint8; CD_VBATTERY_EXTREMELY_HIGH parameter uint8; CD_VBATTERY_DEBOUNCE_EXTREMELY_HIGH parameter uint16; HIGH parameter uint8 =10; OORL parameter uint8 =22; LOW parameter uint8 =9; NORMAL parameter uint8 =8; EXTREMELY_LOW parameter uint8 =14; EXTREMELY_HIGH parameter uint8 =11; ENGINE_CRANKING parameter uint8 =2; NON_FUNCTIONAL parameter uint8 =255; CD_VOLTAGE_HYSTERESIS parameter fixdt(0,8,4); CD_ALTERNATOR_FUNCTION parameter uint8; CD_ALTERNATOR_HIGH parameter uint8; CD_ALTERNATOR_LOW parameter uint8; state_Alternator output uint8; CD_ALTERNATOR_ALARM_ENGINE_SPEED parameter uint16; flt_EngineSpeed input uint16; CD_ALTERNATOR_DEBOUNCE_HIGH parameter uint16; CD_ALTERNATOR_DEBOUNCE_LOW parameter uint16

== stateflow chart VBattery/LP_Filter_Adj_Gain1/LP_Fitler_Adj_Gain ==
  state INITIAL
    en:Output = Input;
  state LP_FILTER
    du:Output = Output + ((Input - Output)/(1 << Gain));
  (default) -> INITIAL
  INITIAL -> LP_FILTER
  data: Gain input uint8; Input input fixdt(1,16,8); Output output fixdt(1,32,16)
